simulink model "Transf_3f"  (Simulink 4.00)
settings: Solver=ode23tb  StartTime=0.0  StopTime=0.1  MaxStep=1e-3  MinStep=1e-4  RelTol=1e-3
libraries: powerlib_extras x6, powerlib2 x3
settings Model: BlockReductionOpt=off

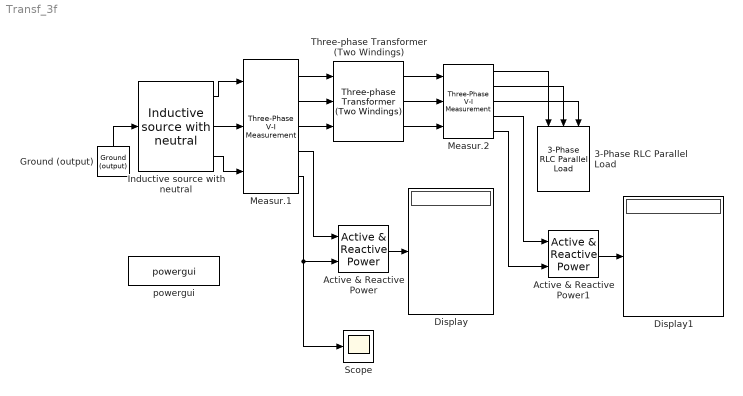
== system Transf_3f ==
  3-Phase RLC Parallel Load : powerlib_extras/Three-Phase Library/3-Phase RLC Parallel Load  Orientation=down  Vpp=380  fn=50  P3=100e3  QL3=50e3  QC3=0
  Active & Reactive Power : powerlib_extras/Measurements/Active & Reactive Power  f1=50
  Active & Reactive Power1 : powerlib_extras/Measurements/Active & Reactive Power  f1=50
  Display : Display
      settings: Format=short
  Display1 : Display
      settings: Format=short
  Ground (output) : powerlib2/Connectors/Ground (output)  Tag=PoWeRsYsTeMbLoCk  Orientation=up  PSBOutputType=1
  Inductive source with neutral : powerlib_extras/Three-Phase Library/Inductive source with neutral  V=1000  Phi=0  F=50  R=0.001  L=1e-4
  Measur.1 : powerlib_extras/Measurements/Three-Phase V-I Measurement  Vpu=off  Vbase=500e3  Ppu=off  Pbase=100e6
  Measur.2 : powerlib_extras/Measurements/Three-Phase V-I Measurement  Vpu=off  Vbase=500e3  Ppu=off  Pbase=100e6
  Scope : Scope
      settings: TimeRange=auto  YMin=-5  YMax=5  SaveToWorkspace=off  SaveName=ScopeData  LimitDataPoints=on  MaxDataPoints=5000
  Three-phase Transformer (Two Windings) : powerlib2/Elements/Three-phase Transformer (Two Windings)  Tag=PoWeRsYsTeMbLoCk  nominal=[ 500e3 , 50 ]  type1=Y  params1=[ 660 , 0.02 , 0.8 ]  type2=Y  params2=[ 380 , 0.02 , 0.8 ]  ynsat=off  rmag=500  lm=500  sat="[ 0,0  ;  0.005,1.2  ;  1.0,1.4 ]"  sif=off  phi0=[ 0.8 , -0.8 , 0.7 ]  mesure=None  PSBOutputType=1111
  powergui : powerlib2/powergui  matfilesaved=off  Frange=logspace(0,3,50)  Ylog=off  Xlog=off  save=off  variable=ZData  display=off
  wires:
  Ground (output)/1 -> Inductive source with neutral/1
  Inductive source with neutral/1 -> Measur.1/1
  Measur.1/1 -> Three-phase Transformer (Two Windings)/1
  Measur.1/2 -> Three-phase Transformer (Two Windings)/2
  Measur.1/3 -> Three-phase Transformer (Two Windings)/3
  Inductive source with neutral/2 -> Measur.1/2
  Inductive source with neutral/3 -> Measur.1/3
  Measur.1/5 -> Active & Reactive Power/2, Scope/1
  Measur.1/4 -> Active & Reactive Power/1
  Three-phase Transformer (Two Windings)/1 -> Measur.2/1
  Three-phase Transformer (Two Windings)/2 -> Measur.2/2
  Three-phase Transformer (Two Windings)/3 -> Measur.2/3
  Measur.2/5 -> Active & Reactive Power1/2
  Measur.2/4 -> Active & Reactive Power1/1
  Measur.2/1 -> 3-Phase RLC Parallel Load/1
  Measur.2/2 -> 3-Phase RLC Parallel Load/2
  Measur.2/3 -> 3-Phase RLC Parallel Load/3
  Active & Reactive Power/1 -> Display/1
  Active & Reactive Power1/1 -> Display1/1
